simulink model "lab4_simulink5receiver"  (R2024a)
settings: Solver=VariableStepAuto  StartTime=0.0  StopTime=inf  RelTol=1e-3
undefined symbols (not defined in the file or in its folder): designMultirateFIR
libraries: dspsnks4 x1, dspmlti4 x1, simulink x1
settings Model: SimulationMode=accelerator  Creator=PULLEY  LastModifiedBy=PULLEY

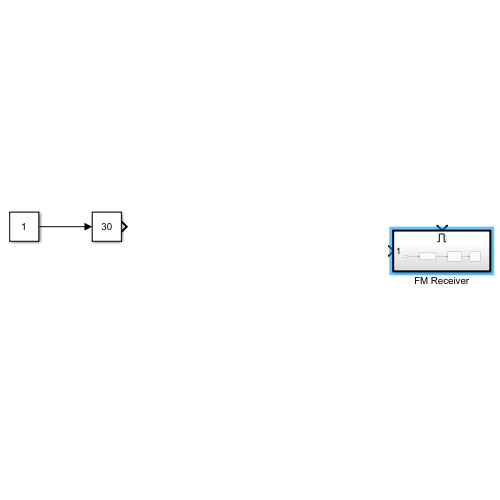
[thumbnail: Simulink's stored preview of the top-level diagram]
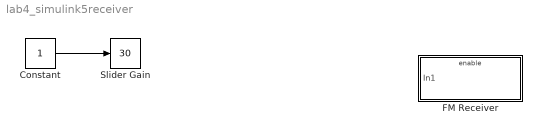
== system lab4_simulink5receiver ==
  Constant : Constant
  FM Receiver : Subsystem
  Slider Gain : simulink/Math Operations/Slider Gain  gain=30  low=0  high=50
  wires:
  Constant/1 -> Slider Gain/1

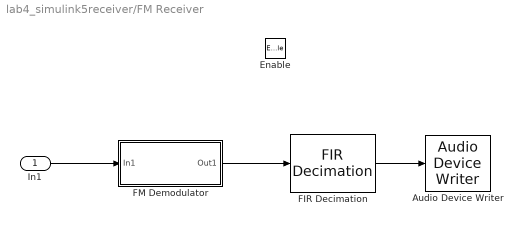
== system lab4_simulink5receiver/FM Receiver ==
  In1 : Inport
  Enable : EnablePort
  Audio Device Writer : dspsnks4/Audio Device Writer  Driver=DirectSound  Device=Default  InheritSampleRate=off  SampleRate=44100  BitDepth=16-bit integer  BufferSize=4096  NumBuffers=10  DefaultOutputChannelMapping=on  OutputChannelMapping=1:2  OutputNumUnderrunSamples=off  DriverIdx=1  DeviceWarnFlag=''
  FIR Decimation : dspmlti4/FIR Decimation  FilterSource=Auto  h=designMultirateFIR(1,2)  D=5  filtStruct=Direct form  FilterObject=FDECIM  framing=Allow multirate processing  AllowArbitraryInputLength=off  inputOffset=0  outputBufInitCond=0  roundingMode=Floor  overflowMode=off  firstCoeffDataTypeStr=Inherit: Same word length as input  firstCoeffMin=[]  firstCoeffMax=[]  firstCoeffLastDataTypeStr=Inherit: Same word length as input  outputDataTypeStr=Inherit: Same as accumulator  outputMin=[]  outputMax=[]  outputLastDataTypeStr=Inherit: Same as accumulator
      settings: LibrarySourceBlock=|
      | dsphdlsupportfiltering/FIR
      | Decimation
  FM Demodulator : Subsystem
  wires:
  In1/1 -> FM Demodulator/1(In1)
  FM Demodulator/1(Out1) -> FIR Decimation/1
  FIR Decimation/1 -> Audio Device Writer/1

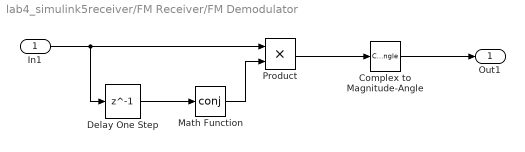
== system lab4_simulink5receiver/FM Receiver/FM Demodulator ==
  In1 : Inport
  Complex to Magnitude-Angle : ComplexToMagnitudeAngle  Output=Angle
  Delay One Step : Delay  DelayLength=1
  Math Function : Math  Operator=conj
  Product : Product
  Out1 : Outport
  wires:
  Delay One Step/1 -> Math Function/1
  In1/1 -> Delay One Step/1, Product/1
  Math Function/1 -> Product/2
  Product/1 -> Complex to Magnitude-Angle/1
  Complex to Magnitude-Angle/1 -> Out1/1
